simulink library "library_ALICAT_FLOW_RW"  (R2024b)
settings: Solver=VariableStepAuto  StartTime=0.0  StopTime=10.0  RelTol=1e-3
undefined symbols (not defined in the file): Controller
settings Model: Creator=GavinWilliamson  LastModifiedBy=GavinWilliamson

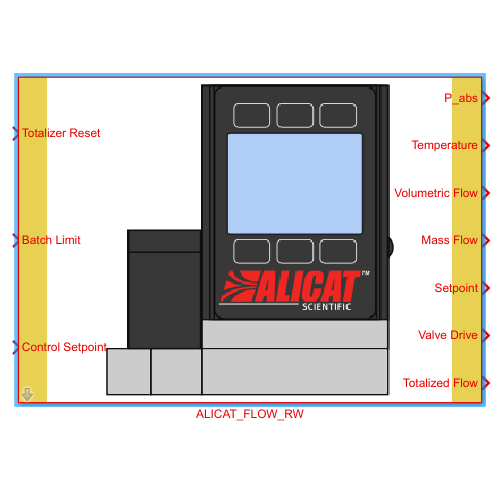
[thumbnail: Simulink's stored preview of the top-level diagram]
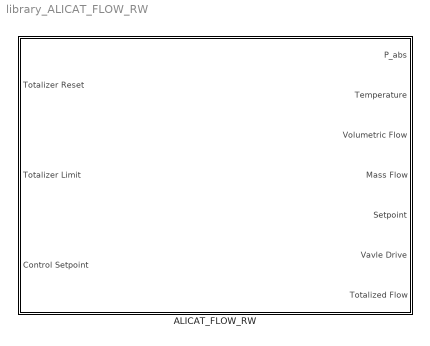
== system library_ALICAT_FLOW_RW ==
  ALICAT_FLOW_RW : Subsystem  mask{Port="COM4", Device_Name='A', gs_type=Hydrogen, dv_typ=Controller, totlzer_sw=on, vlvDR_sw=on, cntrl_sw=on, contrl_typ=Mass Flow, batch_sw=on}
      mask prompts: Device_Name "Device Identifier"; gs_type "Gas Type"; dv_typ "Device Type"; totlzer_sw "Enable Totalizer (*Totalizer Reset command will be functional)"; vlvDR_sw "Enable Valve Drive Recording"; cntrl_sw "Enable ALICAT Controller"; contrl_typ "Setpoint Variable"; batch_sw "Enable Batching"
      mask help: Default Mask
      mask Help: web(which('help_ALICAT_FLOW_RW.html'), '-helpbrowser')
      mask TypeOptions Port:
      | Level-2 MATLAB
      | S-Function/Port
      mask TypeOptions Device_Name:
      | Level-2 MATLAB
      | S-Function/Device_Name
      mask TypeOptions gs_type:
      | Level-2 MATLAB
      | S-Function/gs_type
      mask TypeOptions dv_typ:
      | Level-2 MATLAB
      | S-Function/dv_typ
      mask TypeOptions totlzer_sw:
      | Level-2 MATLAB
      | S-Function/totlzer_sw
      mask TypeOptions vlvDR_sw:
      | Level-2 MATLAB
      | S-Function/vlvDR_sw
      mask TypeOptions cntrl_sw:
      | Level-2 MATLAB
      | S-Function/cntrl_sw
      mask TypeOptions contrl_typ:
      | Level-2 MATLAB
      | S-Function/contrl_typ
      mask TypeOptions batch_sw:
      | Level-2 MATLAB
      | S-Function/batch_sw
      mask DialogControl Container3 Prompt: General
      mask DialogControl DescGroupVar_copy Prompt: ALICAT_RW
      mask DialogControl DescTextVar_copy Prompt: Block controls and reads an ALICAT standard flow meters/controllers over serial communication. Labels on the ports on the block will disappear if there are not valid for the configuration selected. To see all port labels you can look under the mask of this block.
      mask DialogControl Container10 Prompt: Communication Parameters
      mask DialogControl Container11 Prompt: Data Logging Options
      mask DialogControl Container12 Prompt: Control Options
      mask DialogControl Container5 Prompt: Instructions
      mask DialogControl Container6 Prompt: Inputs
      mask DialogControl Control2 Prompt: Totalizer Reset: Input should be a constant block that is set to 0. A push button should be linked to the block to change the value to 1 when pushed. When the button is pushed the totalizer will then be reset.
      mask DialogControl Control3 Prompt: Batch Limit: The input for totalizer limit will only be written to the device if the totalizer and batching are enabled in the register parameters.
      mask DialogControl Container7 Prompt: Register Parameters
      mask DialogControl Container18 Prompt: Communication Parameters
      mask DialogControl Control16 Prompt: Port: Communication port that ALICAT is connected to [string]
      mask DialogControl Control14 Prompt: Device Identifier: Unit ID of ALICAT [char]
      mask DialogControl Container17 Prompt: Gas Type
      mask DialogControl Control15 Prompt: Process gas flowing through ALICAT
      mask DialogControl Container13 Prompt: Device Type
      mask DialogControl Control7 Prompt: Select whether the ALICAT that is connected to the COM Port is a controller or meter. This is important to ensure invalid commands are not sent to the device, and to ensure that the outputted data is in the expected format.
      mask DialogControl Container14 Prompt: Data Logging Options
      mask DialogControl Control6 Prompt: Enable Totalizer: This will enable the totalizer on the ALICAT device, which functions on both controllers and meters. **THE TOTALIZER RESET INPUT WILL BECOME FUNCTIONAL IF THIS IS ENABLED**
      mask DialogControl Control8 Prompt: Enable Valve Drive Recording: This will set the valve drive position to be outputted by an ALICAT controller and will also set the value to display on the screen.
      mask DialogControl Container15 Prompt: Control Options
      mask DialogControl Control9 Prompt: Enable ALICAT Controller: This allows an ALICAT controller to be controlled through Simulink. If unchecked, Simulink will just configure the data logging option parameters and read the device outputs.
      mask DialogControl Container16 Prompt: Setpoint Variable
      mask DialogControl Control10 Prompt: If set to "Valve Drive", "Control Setpoint" should be set to the percentage open on the range of 0-100. Where 0 corresponds to closed and 100 corresponds to fully open.
      mask DialogControl Control11 Prompt: Enable Batching: This enables the batching on the ALICAT and enables the batch limit to be updated while the model is running.
      mask Display:
      | image('AlicatMFCIcon.png', [0,0,0,0,100,100]);
      | 
      | %input ports
      | if strcmp(get_param(gcb,'totlzer_sw'),'on')
      |     port_label('input', 1, 'Totalizer Reset');
      | end
      | if strcmp(get_param(gcb,'batch_sw'),'on')
      |     port_label('input', 2, 'Batch Limit');
      | end
      | if strcmp(get_param(gcb,'cntrl_sw'),'on')
      |     port_label('input', 3, 'Control Setpoint');
      | end
      | 
      | %output ports
      | port_label('output', 1, 'P_abs');
      | port_label('output', 2, 'Temperature');
      | port_label('output', 3, 'Volumetric Flow');
      | port_label('output', 4, 'Mass Flow');
      | if strcmp(get_param(gcb,'dv_typ'),'Controller')
      |     port_label('output', 5, 'Setpoint');
      | end
      | if strcmp(get_param(gcb,'vlvDr_sw'),'on')
      |     port_label('output', 6, 'Valve Drive');
      | end
      | if strcmp(get_param(gcb,'totlzer_sw'),'on')
      |     port_label('output', 7, 'Totalized Flow');
      | end

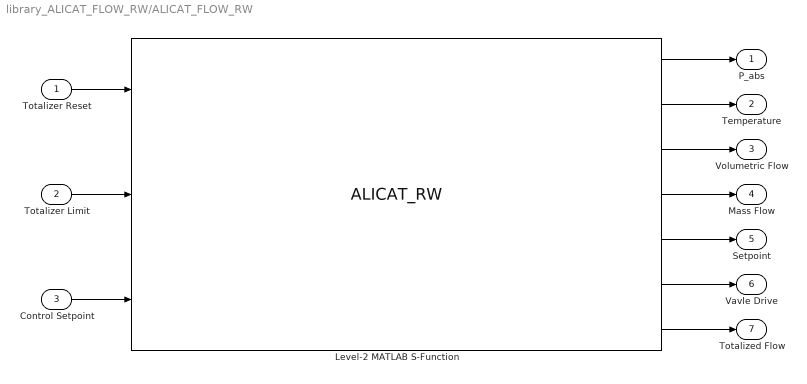
== system library_ALICAT_FLOW_RW/ALICAT_FLOW_RW ==
  Totalizer Reset : Inport
  Totalizer Limit : Inport  Port=2
  Control Setpoint : Inport  Port=3
  Level-2 MATLAB S-Function : M-S-Function  FunctionName=ALICAT_RW  Parameters=Port, Device_Name, gs_type, batch_sw, contrl_typ, cntrl_sw, dv_typ,totlzer_sw,vlvDR_sw  mask{Port=Port, Device_Name=Device_Name, gs_type=Hydrogen, dv_typ=Controller, totlzer_sw=on, vlvDR_sw=on, cntrl_sw=on, contrl_typ=Mass Flow, batch_sw=on}
      mask prompts: Device_Name "Device Identifier"; gs_type "Gas Type"; dv_typ "Device Type"; totlzer_sw "Enable Totalizer"; vlvDR_sw "Enable Valve Drive Recording"; cntrl_sw "Enable ALICAT Controller"; contrl_typ "Setpoint Variable"; batch_sw "Enable Batching"
      mask TypeOptions gs_type: Hydrogen | Nitrogen | Air
      mask TypeOptions dv_typ: Controller | Meter
      mask TypeOptions contrl_typ: Mass Flow | Volumetric Flow | Absolute Pressure | Valve Drive
      mask DialogControl DescGroupVar Prompt: ALICAT_RW
      mask DialogControl DescTextVar Prompt: *See mask of subsystem
      mask DialogControl Container4 Prompt: Connection Parameters
      mask DialogControl Container5 Prompt: Data Logging Options
      mask DialogControl Container6 Prompt: Control Options
      mask Display:
      | image('AlicatMFCIcon.png');
      | 
      | 
      | port_label('input', 1, 'Totalizer Reset');
      | port_label('input', 2, 'Totalizer Limit');
      | port_label('input', 3, 'Control Setpoint');
      | 
      | port_label('output', 1, 'P_abs');
      | port_label('output', 2, 'Temperature');
      | port_label('output', 3, 'Volumetric Flow');
      | port_label('output', 4, 'Mass Flow');
      | port_label('output', 5, 'Setpoint');
      | port_label('output', 6, 'Valve Drive');
      | port_label('output', 7, 'Totalized Flow');
  P_abs : Outport
  Temperature : Outport  Port=2
  Volumetric Flow : Outport  Port=3
  Mass Flow : Outport  Port=4
  Setpoint : Outport  Port=5
  Vavle Drive : Outport  Port=6
  Totalized Flow : Outport  Port=7
  wires:
  Control Setpoint/1 -> Level-2 MATLAB S-Function/3
  Totalizer Limit/1 -> Level-2 MATLAB S-Function/2
  Totalizer Reset/1 -> Level-2 MATLAB S-Function/1
  Level-2 MATLAB S-Function/1 -> P_abs/1
  Level-2 MATLAB S-Function/2 -> Temperature/1
  Level-2 MATLAB S-Function/3 -> Volumetric Flow/1
  Level-2 MATLAB S-Function/4 -> Mass Flow/1
  Level-2 MATLAB S-Function/5 -> Setpoint/1
  Level-2 MATLAB S-Function/7 -> Totalized Flow/1
  Level-2 MATLAB S-Function/6 -> Vavle Drive/1
